simulink model "mseCaseMuxOfTwo"  (R2024b)
settings: Solver=VariableStepAuto  StartTime=0.0  StopTime=10.0  RelTol=1e-3
settings Model: Creator=DarianMuresan  LastModifiedBy=ferbe
settings RTWCC: GPUComputeCapability=3.5

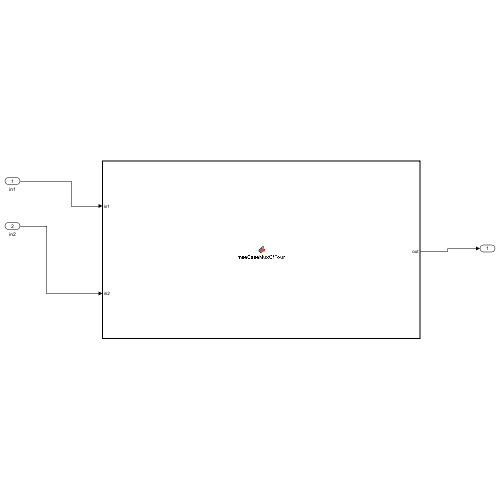
[thumbnail: Simulink's stored preview of the top-level diagram]
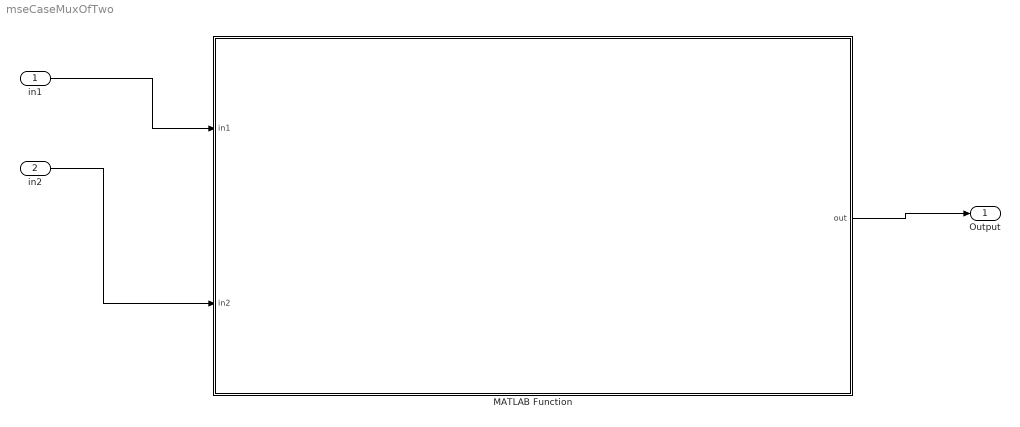
== system mseCaseMuxOfTwo ==
  in1 : Inport
  in2 : Inport  Port=2
  MATLAB Function : MATLAB Function  TreatAsAtomicUnit=on
  Output : Outport
  wires:
  in2/1 -> MATLAB Function/2(in2)
  in1/1 -> MATLAB Function/1(in1)
  MATLAB Function/1(out) -> Output/1

== matlab function mseCaseMuxOfTwo/MATLAB Function ==
  data: in1 input; out output; in2 input
function out = mseCaseMuxOfFour(in1,in2)

% Method to mux 4 inputs into one of 4 possible outputs based on
% the first non-negative input.  To be paired with CaseSplitOfFour.
%
% Written by: Darian Muresan
% Last Modified: 10/10/2024

if nargin<2
    in2=-1;
end

if in1>=0
    out = in1;
elseif in2>=0
    out = in2;
else
    out = -1;
end
